simulink library "MCopter"  (R2015a)
settings: Solver=ode45  StartTime=0.0  StopTime=10.0  RelTol=1e-3
undefined symbols (not defined in the file or in its folder): a, C_d0, h, inertia_switch, J_T, Newton, Omega_TTO, R, Raphson, rho, sigma, theta_0, theta_1, Throtle_TTO, Torque_TTO, v_i0, v_i_adim, Vx_adim, Vz_adim
undefined symbols (not defined in the file): Initial_Omegas, Initial_Torques, l, Rotation_sign, Tau_motors
libraries: MCopter x6, vrlib x3, aerolibutil x3
settings Model: Creator=David  LastModifiedBy=David
settings OptimizationCC: ExpressionDepthLimit=2147483647
settings DebuggingCC: UnderspecifiedInitializationDetection=Classic  MergeDetectMultiDrivingBlocksExec=none  SolverPrmCheckMsg=warning  StateNameClashWarn=warning

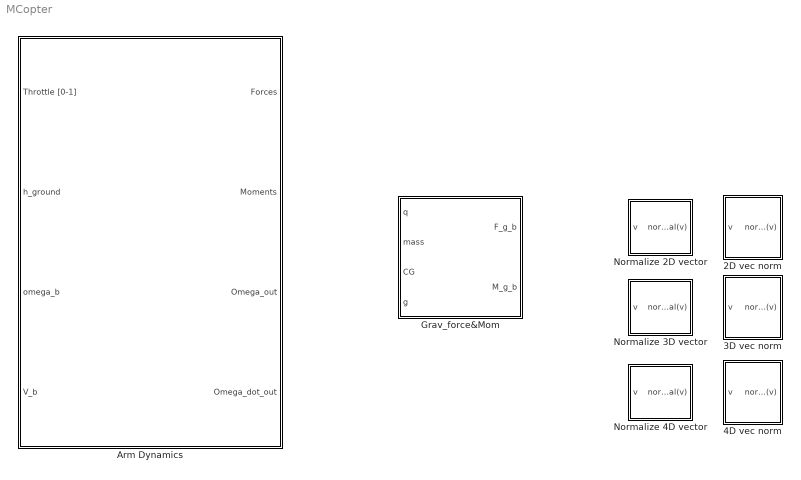
== system MCopter ==
  2D vec norm : Subsystem  TreatAsAtomicUnit=on
  3D vec norm : Subsystem  TreatAsAtomicUnit=on
  4D vec norm : Subsystem  TreatAsAtomicUnit=on
  Arm Dynamics : Subsystem  TreatAsAtomicUnit=on  mask(Arm dynamics, forces and moments){Rot_sign=Rotation_sign(1), arm_num=1, tau=Tau_motors, arm_hub_pos=l*[1;0;0], J_T=J_T, h=h, Torq_ini=Initial_Torques(1), Omega_ini=Initial_Omegas(1)}
      mask prompts: Rot_sign "Rotation Sign"; arm_num "Arm number"; tau "Tau motors"; arm_hub_pos "Arm Hub position"; J_T "Inertia Motor+Prop"; h "h propeller hub"; Torq_ini "Torque Initial Condition"; Omega_ini "Omega Initial Condition"
      mask help:
      | Author: David Torres
      |
      | This block assumes that the spinning axis of the propellers is the same axis as the z-axis of the vehicle.
      mask TypeOptions Rot_sign: Aerodynamics Propeller/Rot_sign
      mask TypeOptions tau: ESC+Motor Dynamcis/tau
      mask TypeOptions arm_hub_pos: Hub_position/Value
      mask TypeOptions J_T: ESC+Motor Dynamcis/J_T
      mask TypeOptions h: h arm/Value
      mask TypeOptions Torq_ini: Initial_torque/X0
      mask TypeOptions Omega_ini: initial_omega/X0 | omega_ini/Value
      mask Display:
      | % fprintf(' Arm number %i \n dynamics',arm_num)
      | 
      | 
      | disp(['{\bf \fontsize{16}',sprintf('Arm number\n\n'),num2str(arm_num),sprintf('\n\n Dynamics '),'}'], 'texmode','on');
  Grav_force&Mom : Subsystem  TreatAsAtomicUnit=on
  Normalize 2D vector : Subsystem  TreatAsAtomicUnit=on
  Normalize 3D vector : Subsystem  TreatAsAtomicUnit=on
  Normalize 4D vector : Subsystem  TreatAsAtomicUnit=on

== system MCopter/2D vec norm ==
  v : Inport
  norm^2rm : Subsystem  TreatAsAtomicUnit=on
  sqrt : Sqrt  AlgorithmType=Newton-Raphson  SaturateOnIntegerOverflow=on
  norm(v) : Outport
  wires:
  sqrt/1 -> norm(v)/1
  norm^2rm/1(norm(v)) -> sqrt/1
  v/1 -> norm^2rm/1(v)

== system MCopter/3D vec norm ==
  v : Inport
  norm^2rm : Subsystem  TreatAsAtomicUnit=on
  sqrt : Sqrt  AlgorithmType=Newton-Raphson  SaturateOnIntegerOverflow=on
  norm(v) : Outport
  wires:
  v/1 -> norm^2rm/1(v)
  norm^2rm/1(norm(v)) -> sqrt/1
  sqrt/1 -> norm(v)/1

== system MCopter/4D vec norm ==
  v : Inport
  norm^2rm : Subsystem  TreatAsAtomicUnit=on
  sqrt : Sqrt  AlgorithmType=Newton-Raphson  SaturateOnIntegerOverflow=on
  norm(v) : Outport
  wires:
  sqrt/1 -> norm(v)/1
  norm^2rm/1(norm(v)) -> sqrt/1
  v/1 -> norm^2rm/1(v)

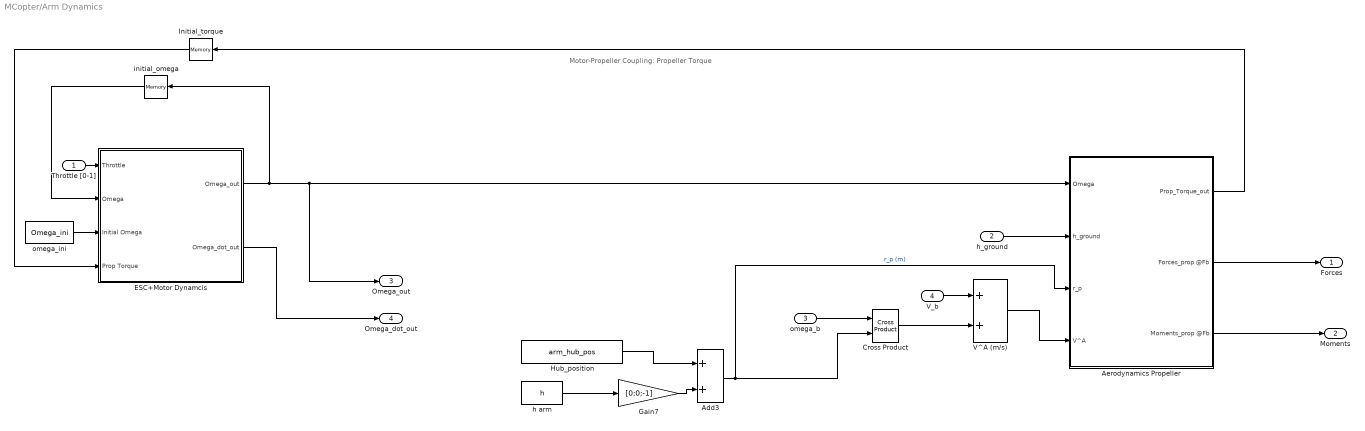
== system MCopter/Arm Dynamics ==
  note: Motor-Propeller Coupling: Propeller Torque
  Throttle [0-1] : Inport
  h_ground : Inport  Port=2
  omega_b : Inport  Port=3
  V_b : Inport  Port=4
  Add3 : Sum
  Aerodynamics Propeller : Subsystem  TreatAsAtomicUnit=on  mask{Rot_sign=Rot_sign}
      mask prompts: Rot_sign "Rotation Sign"
      settings: MinAlgLoopOccurrences=on
      mask TypeOptions Rot_sign: Rotation_sign/Value
  Cross Product : vrlib/Utilities/Cross Product
  ESC+Motor Dynamcis : Subsystem  TreatAsAtomicUnit=on  VariantControl=Variant_completed  mask{Inertia_swithc_var=Motor+Prop, J_T=J_T, tau=tau}
      mask prompts: Inertia_swithc_var "Which inertia to use?"; J_T "Inertia Motor+Prop"; tau "Tau motors"
      mask TypeOptions Inertia_swithc_var: None | Motor+Prop
      mask Callback Inertia_swithc_var:
      | val = get_param(gcb,'MaskValues');
      | % lower(val{1})
      | switch lower(val{1})
      |  case {'none'}
      |   inertia_switch=1;
      |  case {'motor+prop'}
      |   inertia_switch=2;
      | end
      mask TypeOptions J_T: Inertia of prop+motor/Value
      mask TypeOptions tau: Time constant motors/Value
  Gain7 : Gain  Gain=[0;0;-1]
  Hub_position : Constant  Value=arm_hub_pos
  Initial_torque : Memory  X0=Torq_ini
  V^A (m/s) : Sum
  h arm : Constant  Value=h
  initial_omega : Memory  X0=Omega_ini
  omega_ini : Constant  Value=Omega_ini
  Forces : Outport
  Moments : Outport  Port=2
  Omega_out : Outport  Port=3
  Omega_dot_out : Outport  Port=4
  wires:
  Throttle [0-1]/1 -> ESC+Motor Dynamcis/1(Throttle)
  omega_ini/1 -> ESC+Motor Dynamcis/3(Initial Omega)
  ESC+Motor Dynamcis/2(Omega_dot_out) -> Omega_dot_out/1
  ESC+Motor Dynamcis/1(Omega_out) -> initial_omega/1, Omega_out/1, Aerodynamics Propeller/1(Omega)
  h_ground/1 -> Aerodynamics Propeller/2(h_ground)
  omega_b/1 -> Cross Product/1
  Cross Product/1 -> V^A (m/s)/2
  V_b/1 -> V^A (m/s)/1
  V^A (m/s)/1 -> Aerodynamics Propeller/4(V^A)
  Aerodynamics Propeller/2(Forces_prop @Fb) -> Forces/1
  Aerodynamics Propeller/3(Moments_prop @Fb) -> Moments/1
  Aerodynamics Propeller/1(Prop_Torque_out) -> Initial_torque/1
  initial_omega/1 -> ESC+Motor Dynamcis/2(Omega)
  Gain7/1 -> Add3/2
  Hub_position/1 -> Add3/1
  h arm/1 -> Gain7/1
  Add3/1 -> Aerodynamics Propeller/3(r_p), Cross Product/2  "r_p (m)"
  Initial_torque/1 -> ESC+Motor Dynamcis/4(Prop Torque)

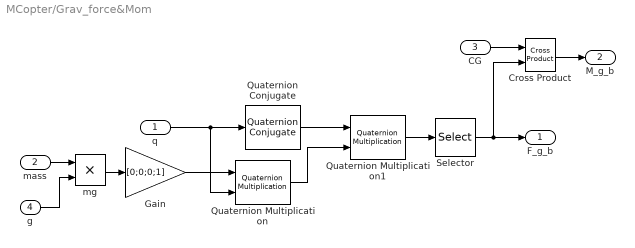
== system MCopter/Grav_force&Mom ==
  q : Inport
  mass : Inport  Port=2
  CG : Inport  Port=3
  g : Inport  Port=4
  Cross Product : vrlib/Utilities/Cross Product
  Gain : Gain  Gain=[0;0;0;1]
  Quaternion Conjugate : aerolibutil/Quaternion Conjugate
  Quaternion Multiplication : aerolibutil/Quaternion Multiplication
  Quaternion Multiplication1 : aerolibutil/Quaternion Multiplication
  Selector : Selector  IndexMode=Zero-based  InputPortWidth=4  Indices=[1:3]
  mg : Product  RndMeth=Zero
  F_g_b : Outport
  M_g_b : Outport  Port=2
  wires:
  mass/1 -> mg/1
  g/1 -> mg/2
  mg/1 -> Gain/1
  Gain/1 -> Quaternion Multiplication/1
  q/1 -> Quaternion Conjugate/1, Quaternion Multiplication/2
  Quaternion Conjugate/1 -> Quaternion Multiplication1/1
  Quaternion Multiplication/1 -> Quaternion Multiplication1/2
  Quaternion Multiplication1/1 -> Selector/1
  Selector/1 -> Cross Product/2, F_g_b/1
  CG/1 -> Cross Product/1
  Cross Product/1 -> M_g_b/1

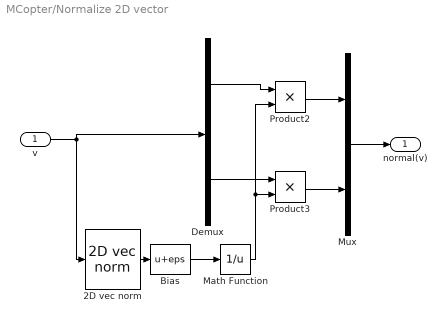
== system MCopter/Normalize 2D vector ==
  v : Inport
  2D vec norm : MCopter/2D vec norm
  Bias : Bias  Bias=eps
  Demux : Demux  Outputs=2
  Math Function : Math  Operator=reciprocal  SaturateOnIntegerOverflow=on
  Mux : Mux  Inputs=2
  Product2 : Product  Inputs=**
  Product3 : Product  Inputs=**
  normal(v) : Outport
  wires:
  Math Function/1 -> Product2/2, Product3/2
  Demux/2 -> Product3/1
  Demux/1 -> Product2/1
  Mux/1 -> normal(v)/1
  v/1 -> 2D vec norm/1, Demux/1
  Bias/1 -> Math Function/1
  Product2/1 -> Mux/1
  Product3/1 -> Mux/2
  2D vec norm/1 -> Bias/1

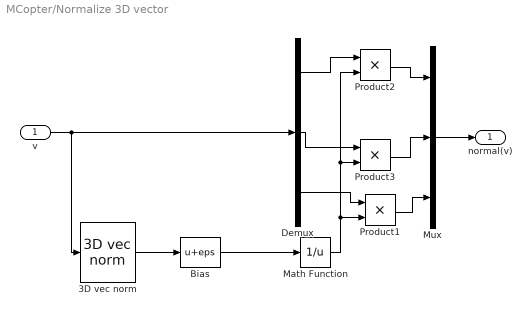
== system MCopter/Normalize 3D vector ==
  v : Inport
  3D vec norm : MCopter/3D vec norm
  Bias : Bias  Bias=eps
  Demux : Demux  Outputs=3
  Math Function : Math  Operator=reciprocal  SaturateOnIntegerOverflow=on
  Mux : Mux  Inputs=3
  Product1 : Product  Inputs=**
  Product2 : Product  Inputs=**
  Product3 : Product  Inputs=**
  normal(v) : Outport
  wires:
  Demux/2 -> Product3/1
  Demux/1 -> Product2/1
  Mux/1 -> normal(v)/1
  v/1 -> 3D vec norm/1, Demux/1
  3D vec norm/1 -> Bias/1
  Product2/1 -> Mux/1
  Product3/1 -> Mux/2
  Demux/3 -> Product1/1
  Math Function/1 -> Product2/2, Product3/2, Product1/2
  Product1/1 -> Mux/3
  Bias/1 -> Math Function/1

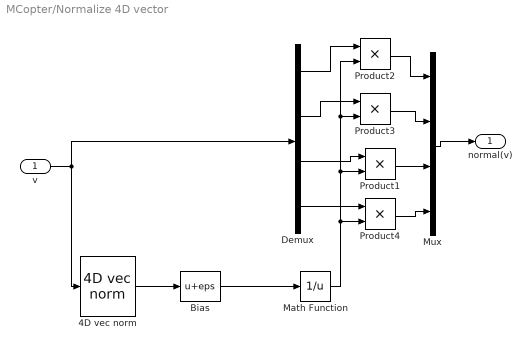
== system MCopter/Normalize 4D vector ==
  v : Inport
  4D vec norm : MCopter/4D vec norm
  Bias : Bias  Bias=eps
  Demux : Demux
  Math Function : Math  Operator=reciprocal  SaturateOnIntegerOverflow=on
  Mux : Mux
  Product{1..4} (4 alike) : Product  Inputs=**
  normal(v) : Outport
  wires:
  Bias/1 -> Math Function/1
  Product1/1 -> Mux/3
  Math Function/1 -> Product4/2, Product1/2, Product3/2, Product2/2
  Demux/3 -> Product1/1
  Product3/1 -> Mux/2
  Product2/1 -> Mux/1
  4D vec norm/1 -> Bias/1
  v/1 -> 4D vec norm/1, Demux/1
  Mux/1 -> normal(v)/1
  Demux/1 -> Product2/1
  Demux/2 -> Product3/1
  Demux/4 -> Product4/1
  Product4/1 -> Mux/4

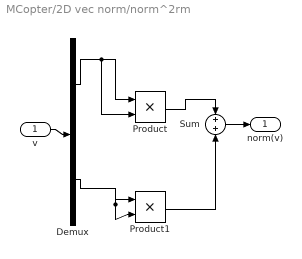
== system MCopter/2D vec norm/norm^2rm ==
  v : Inport
  Demux : Demux  Outputs=2
  Product : Product
  Product1 : Product
  Sum : Sum  Inputs=2
  norm(v) : Outport
  wires:
  v/1 -> Demux/1
  Sum/1 -> norm(v)/1
  Product/1 -> Sum/1
  Product1/1 -> Sum/2
  Demux/1 -> Product/1, Product/2
  Demux/2 -> Product1/2, Product1/1

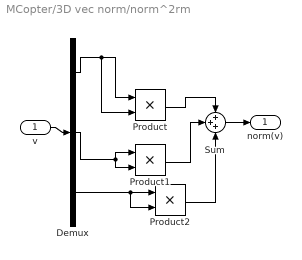
== system MCopter/3D vec norm/norm^2rm ==
  v : Inport
  Demux : Demux  Outputs=3
  Product : Product
  Product1 : Product
  Product2 : Product
  Sum : Sum  Inputs=3
  norm(v) : Outport
  wires:
  Demux/2 -> Product1/2, Product1/1
  Demux/1 -> Product/2, Product/1
  Product1/1 -> Sum/2
  Product/1 -> Sum/1
  Sum/1 -> norm(v)/1
  v/1 -> Demux/1
  Demux/3 -> Product2/2, Product2/1
  Product2/1 -> Sum/3

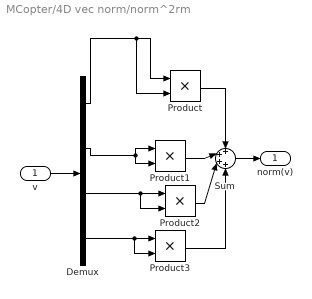
== system MCopter/4D vec norm/norm^2rm ==
  v : Inport
  Demux : Demux
  Product{,1..3} (4 alike) : Product
  Sum : Sum  Inputs=4
  norm(v) : Outport
  wires:
  Product2/1 -> Sum/3
  Demux/3 -> Product2/1, Product2/2
  v/1 -> Demux/1
  Sum/1 -> norm(v)/1
  Product/1 -> Sum/1
  Product1/1 -> Sum/2
  Demux/1 -> Product/1, Product/2
  Demux/2 -> Product1/1, Product1/2
  Demux/4 -> Product3/2, Product3/1
  Product3/1 -> Sum/4

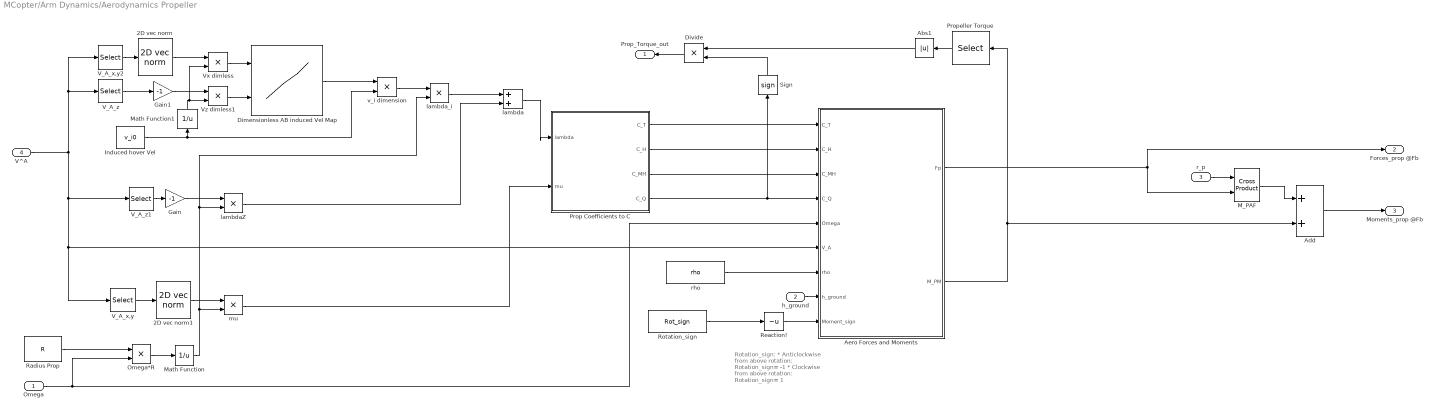
== system MCopter/Arm Dynamics/Aerodynamics Propeller ==
  note: Rotation_sign:
      |
      | * Anticlockwise from above rotation: Rotation_sign= -1
      | * Clockwise from above rotation: Rotation_sign= 1
  Omega : Inport
  h_ground : Inport  Port=2
  r_p : Inport  Port=3
  V^A : Inport  Port=4
  2D vec norm : MCopter/2D vec norm
  2D vec norm1 : MCopter/2D vec norm
  Abs1 : Abs
  Add : Sum
  "Aero Forces and Moments " : Subsystem  TreatAsAtomicUnit=on
  Dimensionless AB induced Vel Map : Lookup_n-D  BreakpointsForDimension1=Vx_adim  BreakpointsForDimension2=Vz_adim  BreakpointsForDimension3=[5, 7]  Table=v_i_adim  TableDataTypeStr=single  IntermediateResultsDataTypeStr=single  ExtrapMethod=Clip  RemoveProtectionInput=on  OutDataTypeStr=single  RndMeth=Zero  FractionDataTypeStr=single  InputSameDT=on
  Divide : Product  Inputs=**
  Gain : Gain  Gain=-1
  Gain1 : Gain  Gain=-1
  Induced hover Vel : Constant  Value=v_i0
  M_PAF : vrlib/Utilities/Cross Product
  Math Function : Math  Operator=reciprocal  SaturateOnIntegerOverflow=on
  Math Function1 : Math  Operator=reciprocal  SaturateOnIntegerOverflow=on
  Omega*R : Product  Inputs=**
  Prop Coefficients to C : MATLAB Function  TreatAsAtomicUnit=on
  Propeller Torque : Selector  IndexMode=Zero-based  InputPortWidth=3  Indices=2
  Radius Prop : Constant  Value=R
  Reaction! : UnaryMinus
  Rotation_sign : Constant  Value=Rot_sign
  Sign : Signum
  V_A_x,y : Selector  IndexMode=Zero-based  InputPortWidth=3  Indices=[0,1]
  V_A_x,y2 : Selector  IndexMode=Zero-based  InputPortWidth=3  Indices=[0,1]
  V_A_z : Selector  IndexMode=Zero-based  InputPortWidth=3  Indices=2
  V_A_z1 : Selector  IndexMode=Zero-based  InputPortWidth=3  Indices=2
  Vx dimless : Product  Inputs=**
  Vz dimless1 : Product  Inputs=**
  lambda : Sum
  lambdaZ : Product  Inputs=**
  lambda_i : Product  Inputs=**
  mu : Product  Inputs=**
  rho : Constant  Value=rho
  v_i dimension : Product  Inputs=**
  Prop_Torque_out : Outport
  Forces_prop @Fb : Outport  Port=2
  Moments_prop @Fb : Outport  Port=3
  wires:
  Radius Prop/1 -> Omega*R/1
  V_A_x,y/1 -> 2D vec norm1/1
  2D vec norm1/1 -> mu/1
  Omega*R/1 -> Math Function/1
  Vx dimless/1 -> Dimensionless AB induced Vel Map/1
  V_A_x,y2/1 -> 2D vec norm/1
  Vz dimless1/1 -> Dimensionless AB induced Vel Map/2
  V_A_z/1 -> Gain1/1
  Induced hover Vel/1 -> v_i dimension/2, Math Function1/1
  Dimensionless AB induced Vel Map/1 -> v_i dimension/1
  v_i dimension/1 -> lambda_i/1
  V_A_z1/1 -> Gain/1
  Gain/1 -> lambdaZ/1
  lambda_i/1 -> lambda/1
  lambdaZ/1 -> lambda/2
  Gain1/1 -> Vz dimless1/1
  lambda/1 -> Prop Coefficients to C/1(lambda)
  Prop Coefficients to C/1(C_T) -> "Aero Forces and Moments "/1(C_T)
  Prop Coefficients to C/2(C_H) -> "Aero Forces and Moments "/2(C_H)
  Prop Coefficients to C/3(C_MH) -> "Aero Forces and Moments "/3(C_MH)
  V^A/1 -> V_A_z1/1, V_A_x,y/1, "Aero Forces and Moments "/6(V_A), V_A_x,y2/1, V_A_z/1
  Omega/1 -> "Aero Forces and Moments "/5(Omega), Omega*R/2
  Add/1 -> Moments_prop @Fb/1
  h_ground/1 -> "Aero Forces and Moments "/8(h_ground)
  Rotation_sign/1 -> Reaction!/1
  "Aero Forces and Moments "/1(Fp) -> M_PAF/2, Forces_prop @Fb/1
  r_p/1 -> M_PAF/1
  M_PAF/1 -> Add/1
  "Aero Forces and Moments "/2("M_PM ") -> Propeller Torque/1, Add/2
  2D vec norm/1 -> Vx dimless/1
  mu/1 -> Prop Coefficients to C/2(mu)
  Prop Coefficients to C/4(C_Q) -> Sign/1, "Aero Forces and Moments "/4(C_Q)
  Reaction!/1 -> "Aero Forces and Moments "/9(Moment_sign)
  Math Function/1 -> mu/2, lambdaZ/2, lambda_i/2
  Math Function1/1 -> Vz dimless1/2, Vx dimless/2
  rho/1 -> "Aero Forces and Moments "/7(rho)
  Divide/1 -> Prop_Torque_out/1
  Propeller Torque/1 -> Abs1/1
  Sign/1 -> Divide/2
  Abs1/1 -> Divide/1

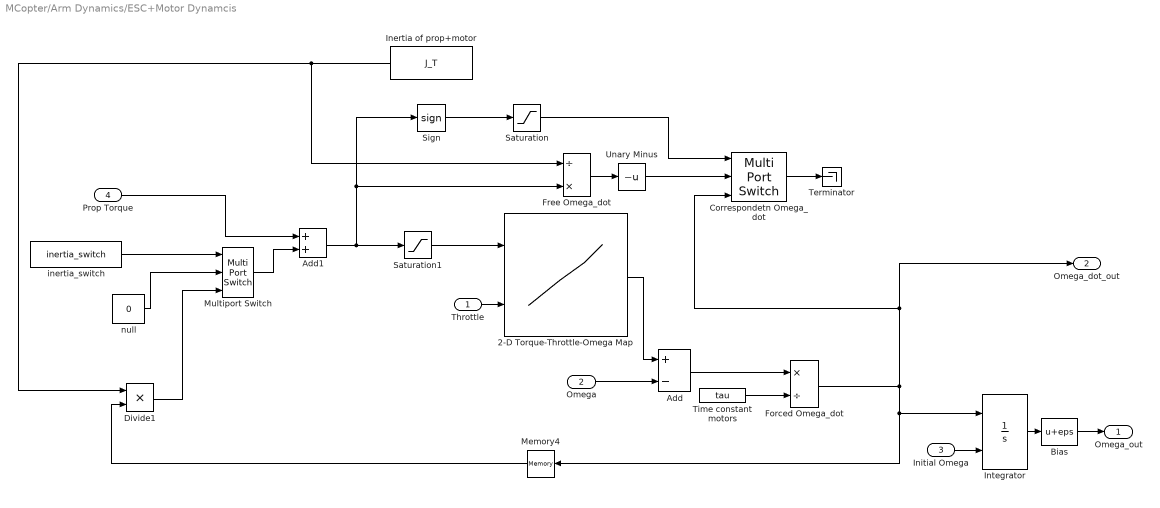
== system MCopter/Arm Dynamics/ESC+Motor Dynamcis ==
  Throttle : Inport
  Omega : Inport  Port=2
  Initial Omega : Inport  Port=3
  Prop Torque : Inport  Port=4
  2-D Torque-Throttle-Omega Map : Lookup_n-D  BreakpointsForDimension1=Torque_TTO(:,1)  BreakpointsForDimension2=Throtle_TTO(1,:)  Table=Omega_TTO  ExtrapMethod=Clip  DiagnosticForOutOfRangeInput=Warning  RemoveProtectionInput=on  RndMeth=Simplest  InputSameDT=on
  Add : Sum  Inputs=+-
  Add1 : Sum
  Bias : Bias  Bias=eps
  Correspondetn Omega_dot : MultiPortSwitch  DataPortOrder=Zero-based contiguous  Inputs=2
  Divide1 : Product  Inputs=**
  Forced Omega_dot : Product  Inputs=*/
  Free Omega_dot : Product  Inputs=/*
  Inertia of prop+motor : Constant  Value=J_T
  Integrator : Integrator  InitialConditionSource=external
  Memory4 : Memory
  Multiport Switch : MultiPortSwitch  Inputs=2
  Saturation : Saturate  UpperLimit=1  LowerLimit=0
  Saturation1 : Saturate  UpperLimit=inf  LowerLimit=0
  Sign : Signum
  Terminator : Terminator
  Time constant motors : Constant  Value=tau
  Unary Minus : UnaryMinus
  inertia_switch : Constant  Value=inertia_switch
  null : Constant  Value=0
  Omega_out : Outport
  Omega_dot_out : Outport  Port=2
  wires:
  Bias/1 -> Omega_out/1
  Divide1/1 -> Multiport Switch/3
  inertia_switch/1 -> Multiport Switch/1
  Memory4/1 -> Divide1/2
  Integrator/1 -> Bias/1
  Forced Omega_dot/1 -> Correspondetn Omega_dot/3, Omega_dot_out/1, Integrator/1, Memory4/1
  Add1/1 -> Sign/1, Free Omega_dot/2, Saturation1/1
  Throttle/1 -> 2-D Torque-Throttle-Omega Map/2
  null/1 -> Multiport Switch/2
  Inertia of prop+motor/1 -> Free Omega_dot/1, Divide1/1
  Multiport Switch/1 -> Add1/2
  Initial Omega/1 -> Integrator/2
  Time constant motors/1 -> Forced Omega_dot/2
  Add/1 -> Forced Omega_dot/1
  Omega/1 -> Add/2
  2-D Torque-Throttle-Omega Map/1 -> Add/1
  Prop Torque/1 -> Add1/1
  Free Omega_dot/1 -> Unary Minus/1
  Saturation/1 -> Correspondetn Omega_dot/1
  Sign/1 -> Saturation/1
  Unary Minus/1 -> Correspondetn Omega_dot/2
  Saturation1/1 -> 2-D Torque-Throttle-Omega Map/1
  Correspondetn Omega_dot/1 -> Terminator/1

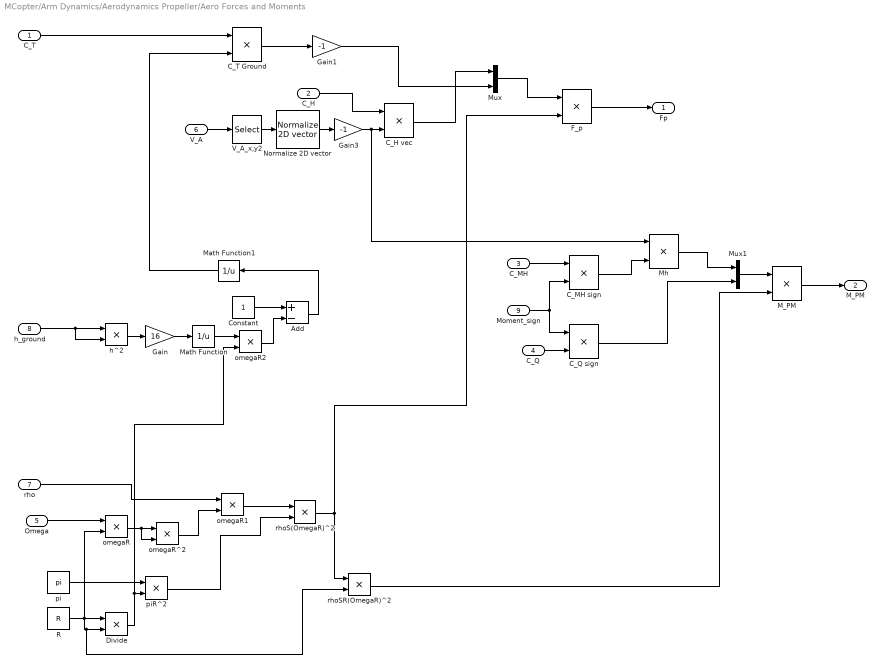
== system MCopter/Arm Dynamics/Aerodynamics Propeller/Aero Forces and Moments  ==
  C_T : Inport
  C_H : Inport  Port=2
  C_MH : Inport  Port=3
  C_Q : Inport  Port=4
  Omega : Inport  Port=5
  V_A : Inport  Port=6
  rho : Inport  Port=7
  h_ground : Inport  Port=8
  Moment_sign : Inport  Port=9
  Add : Sum  Inputs=+-
  C_H vec : Product  Inputs=**
  C_MH sign : Product  Inputs=**
  C_Q sign : Product  Inputs=**
  C_T Ground : Product  Inputs=**
  Constant : Constant
  Divide : Product  Inputs=**
  F_p : Product  Inputs=**
  Gain : Gain  Gain=16
  Gain1 : Gain  Gain=-1
  Gain3 : Gain  Gain=-1
  M_PM : Product  Inputs=**
  Math Function : Math  Operator=reciprocal  SaturateOnIntegerOverflow=on
  Math Function1 : Math  Operator=reciprocal  SaturateOnIntegerOverflow=on
  Mh : Product  Inputs=**
  Mux : Mux  Inputs=[2,1]
  Mux1 : Mux  Inputs=[2,1]
  Normalize 2D vector : MCopter/Normalize 2D vector
  R : Constant  Value=R
  V_A_x,y2 : Selector  IndexMode=Zero-based  InputPortWidth=3  Indices=[0,1]
  h^2 : Product  Inputs=**
  omegaR : Product  Inputs=**
  omegaR1 : Product  Inputs=**
  omegaR2 : Product  Inputs=**
  omegaR^2 : Product  Inputs=**
  pi : Constant  Value=pi
  piR^2 : Product  Inputs=**
  rhoS(OmegaR)^2 : Product  Inputs=**
  rhoSR(OmegaR)^2 : Product  Inputs=**
  Fp : Outport
  "M_PM " : Outport  Port=2
  wires:
  R/1 -> rhoSR(OmegaR)^2/2, Divide/2, omegaR/2, Divide/1
  pi/1 -> piR^2/1
  Divide/1 -> omegaR2/2, piR^2/2
  Omega/1 -> omegaR/1
  rho/1 -> omegaR1/1
  omegaR/1 -> omegaR^2/2, omegaR^2/1
  omegaR^2/1 -> omegaR1/2
  piR^2/1 -> rhoS(OmegaR)^2/2
  omegaR1/1 -> rhoS(OmegaR)^2/1
  C_T/1 -> C_T Ground/1
  h_ground/1 -> h^2/2, h^2/1
  h^2/1 -> Gain/1
  Gain/1 -> Math Function/1
  Math Function/1 -> omegaR2/1
  Constant/1 -> Add/1
  omegaR2/1 -> Add/2
  Add/1 -> Math Function1/1
  Math Function1/1 -> C_T Ground/2
  C_T Ground/1 -> Gain1/1
  V_A_x,y2/1 -> Normalize 2D vector/1
  V_A/1 -> V_A_x,y2/1
  Normalize 2D vector/1 -> Gain3/1
  Gain3/1 -> Mh/1, C_H vec/2
  C_H/1 -> C_H vec/1
  C_H vec/1 -> Mux/1
  Gain1/1 -> Mux/2
  Mux/1 -> F_p/1
  rhoS(OmegaR)^2/1 -> rhoSR(OmegaR)^2/1, F_p/2
  C_MH/1 -> C_MH sign/1
  Moment_sign/1 -> C_MH sign/2, C_Q sign/1
  C_MH sign/1 -> Mh/2
  Mh/1 -> Mux1/1
  F_p/1 -> Fp/1
  Mux1/1 -> M_PM/1
  C_Q/1 -> C_Q sign/2
  C_Q sign/1 -> Mux1/2
  rhoSR(OmegaR)^2/1 -> M_PM/2
  M_PM/1 -> "M_PM "/1

== matlab function MCopter/Arm Dynamics/Aerodynamics Propeller/Prop Coefficients to C ==
  data: lambda input; C_T output; mu input; C_H output; C_MH output; C_Q output; sigma parameter; C_d0 parameter; a parameter; theta_0 parameter; theta_1 parameter
function [C_T,C_H,C_MH,C_Q] = Aero_coeff(lambda,mu, sigma, C_d0, a, theta_0, theta_1)


C_T = sigma*a/4*(theta_0*(2/3+mu^2) +theta_1/2*(1+mu^2) -  lambda );
C_Q =    +sigma*a/4*( 2/3*theta_0 - lambda + theta_1/2)*lambda + sigma*C_d0/8*(1+mu^2);   % Always positive!!!


C_H= sigma*a/4*mu*lambda*(theta_0+theta_1/2) + sigma*C_d0/4*mu; 
C_MH= sigma*a/4*( 2/3*theta_0*mu-1/2*lambda*mu+theta_1*mu/2  );
